simulink model "untitled"  (R2020a)
settings: Solver=FixedStepAuto  StartTime=0.0  StopTime=1  FixedStep=0.00001  RelTol=1e-3
values from neighbouring files (symbols this model uses):
  fp = 1000    [Untitled.m]
  fref = 100    [Untitled.m]
  T = [2 -1 -1;-1 2 -1;-1 -1 2]    [Untitled.m]
  vdc = 300    [Untitled.m]
libraries: simulink x1
settings Model: Creator=ABO-CHIFA  LastModifiedBy=ABO-CHIFA

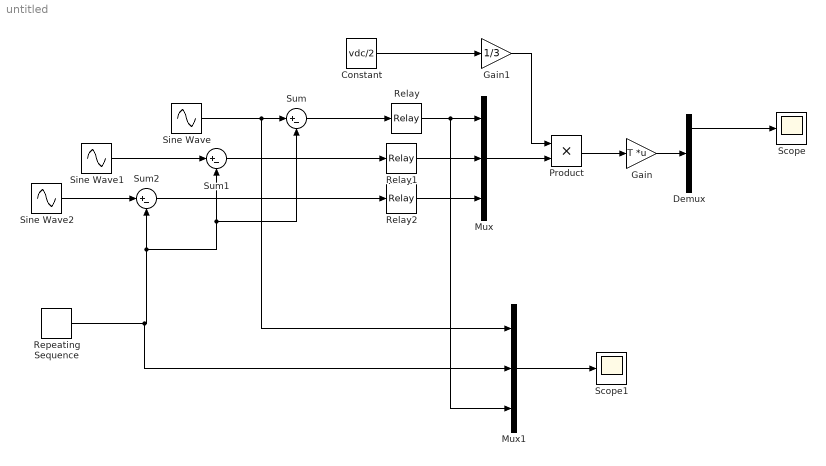
== system untitled ==
  Constant : Constant  Value=vdc/2
  Demux : Demux  Outputs=3
  Gain : Gain  Gain=T  Multiplication=Matrix(K*u)
  Gain1 : Gain  Gain=1/3
  Mux : Mux  Inputs=3
  Mux1 : Mux  Inputs=3
  Product : Product
  Relay : Relay  OnSwitchValue=0.1  OffSwitchValue=-0.1  OffOutputValue=-1
  Relay1 : Relay  OnSwitchValue=0.1  OffSwitchValue=-0.1  OffOutputValue=-1
  Relay2 : Relay  OnSwitchValue=0.1  OffSwitchValue=-0.1  OffOutputValue=-1
  Repeating Sequence : simulink/Sources/Repeating Sequence  rep_seq_t=[0 1/(2*fp) 1/fp]  rep_seq_y=[-1 1 -1]
  Scope : Scope
  Scope1 : Scope
  Sine Wave : Sin  Amplitude=0.8  Frequency=2*pi*fref  SampleTime=0
  Sine Wave1 : Sin  Amplitude=0.8  Frequency=2*pi*fref  Phase=-2*pi/3  SampleTime=0
  Sine Wave2 : Sin  Amplitude=0.8  Frequency=2*pi*fref  Phase=2*pi/3  SampleTime=0
  Sum : Sum  Inputs=|+-
  Sum1 : Sum  Inputs=|+-
  Sum2 : Sum  Inputs=|+-
  wires:
  Mux/1 -> Product/2
  Product/1 -> Gain/1
  Gain1/1 -> Product/1
  Constant/1 -> Gain1/1
  Relay/1 -> Mux1/3, Mux/1
  Relay1/1 -> Mux/2
  Relay2/1 -> Mux/3
  Sum/1 -> Relay/1
  Sum1/1 -> Relay1/1
  Sine Wave/1 -> Mux1/1, Sum/1
  Sine Wave1/1 -> Sum1/1
  Sum2/1 -> Relay2/1
  Sine Wave2/1 -> Sum2/1
  Repeating Sequence/1 -> Mux1/2, Sum/2, Sum1/2, Sum2/2
  Gain/1 -> Demux/1
  Mux1/1 -> Scope1/1
  Demux/1 -> Scope/1
